simulink model "Assignment_2_simulink_2"  (R2025a)
settings: Solver=FixedStepDiscrete  StartTime=0.0  StopTime=inf  FixedStep=0.1  RelTol=1e-3  EnableMultiTasking=on
values from neighbouring files (symbols this model uses):
  Kv = 0.8    [Assignment_2.m]
  tol = 0.05    [Assignment_2.m]
undefined symbols (not defined in the file or in its folder): angular, linear, v_max
libraries: simulink x4, ros2lib x3
settings Model: Creator=nicola-bertocchi  LastModifiedBy=nicola-bertocchi
settings OptimizationCC: DefaultParameterBehavior=Inlined  EnhancedBackFolding=on  PassReuseOutputArgsAs=Individual arguments  ZeroExternalMemoryAtStartup=off  ZeroInternalMemoryAtStartup=off  MaxStackSize=64  OptimizeBlockOrder=speed  DifferentSizesBufferReuse=on  OptimizationCustomize=off  EfficientTunableParamExpr=on
settings DebuggingCC: ParameterTunabilityLossMsg=error
settings HardwareCC: ProdBitPerLong=64.0  ProdHWDeviceType=Intel->x86-64 (Linux 64)
settings SFSimCC: MATLABDynamicMemAlloc=off
settings RTWCC: SystemTargetFile=ert.tlc  HardwareBoard=Robot Operating System 2 (ROS 2)  TLCOptions="-aInlineSetEventsForThisBaseRateFcn=TLC_FALSE -aSuppressMultiTaskScheduler=TLC_FALSE  -aRateBasedStepFcn=0"  TemplateMakefile=ert_default_tmf  Toolchain=Colcon Tools  TargetLang=C++  Description=Embedded Coder
settings CodeAppCC: ForceParamTrailComments=on  IgnoreCustomStorageClasses=off  OperatorAnnotations=on  SimulinkDataObjDesc=on  SFDataObjDesc=on  InsertBlockDesc=on
settings ERTTargetCC: ExtModeTransport=2.0  ExtModeAutomaticAllocSize=off  RootIOFormat=Structure reference  CodeInterfacePackaging=C++ class

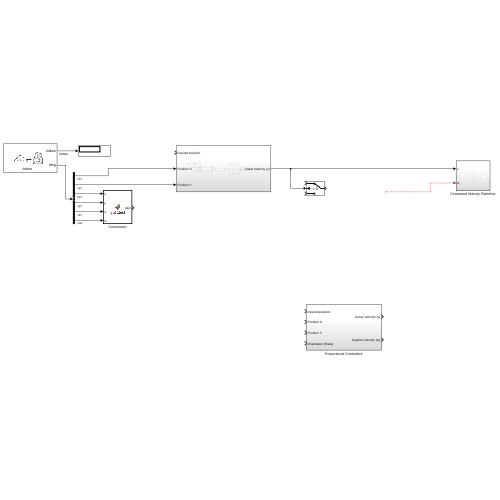
[thumbnail: Simulink's stored preview of the top-level diagram]
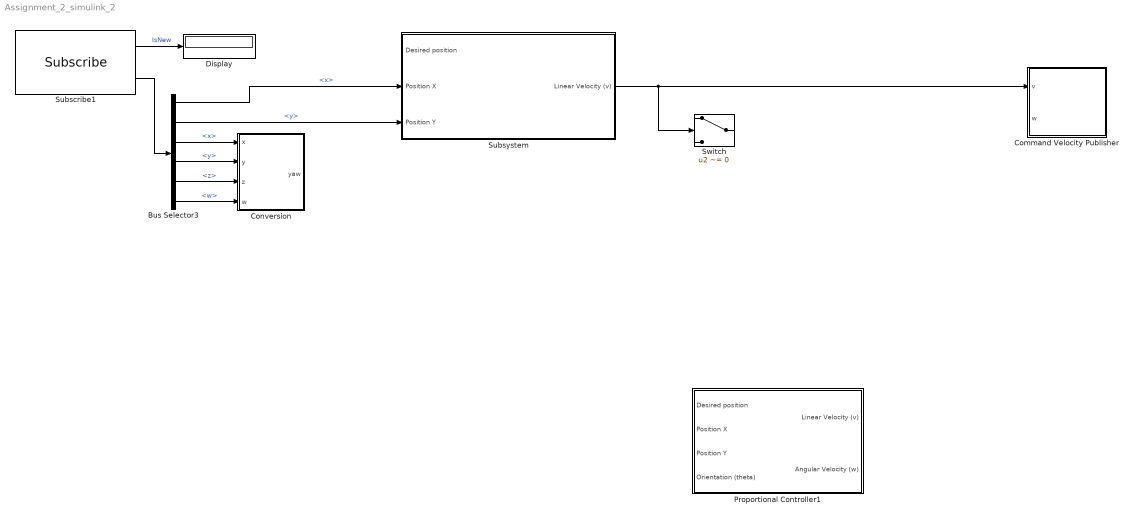
== system Assignment_2_simulink_2 ==
  Bus Selector3 : BusSelector  OutputSignals=pose.pose.position.x,pose.pose.position.y,pose.pose.orientation.x,pose.pose.orientation.y,pose.pose.orientation.z,pose.pose.orientation.w
  Command Velocity Publisher : Subsystem
  Conversion : MATLAB Function  TreatAsAtomicUnit=on
  Display : Display
  Proportional Controller1 : Subsystem
  Subscribe1 : ros2lib/Subscribe  topicSource=Select from ROS network  topic=/odom  messageType=nav_msgs/Odometry  sampleTime=-1  QOSHistory=Keep last  QOSDepth=1  QOSReliability=Reliable  QOSDurability=Volatile  QOSDeadline=Inf  QOSLifespan=Inf  QOSLiveliness=Automatic  QOSLeaseDuration=Inf  QOSAvoidROSNamespaceConventions=off
  Subsystem : Subsystem
  Switch : Switch  Criteria=u2 ~= 0  SaturateOnIntegerOverflow=off  InputSameDT=off
  wires:
  Bus Selector3/6 -> Conversion/4(w)  "<w>"
  Subsystem/1(Linear Velocity (v)) -> Command Velocity Publisher/1(v), Switch/2
  Bus Selector3/1 -> Subsystem/2(Position X)  "<x>"
  Bus Selector3/2 -> Subsystem/3(Position Y)  "<y>"
  Bus Selector3/5 -> Conversion/3(z)  "<z>"
  ? -> Command Velocity Publisher/2(w)
  Subscribe1/2 -> Bus Selector3/1
  Bus Selector3/3 -> Conversion/1(x)  "<x>"
  Bus Selector3/4 -> Conversion/2(y)  "<y>"
  Subscribe1/1 -> Display/1  "IsNew"

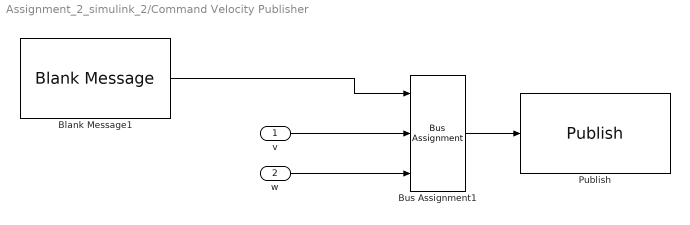
== system Assignment_2_simulink_2/Command Velocity Publisher ==
  v : Inport
  w : Inport  Port=2
  Blank Message1 : ros2lib/Blank Message  messageClass=Message  entityType=geometry_msgs/Twist  messageType=geometry_msgs/Twist  SampleTime=inf
  Bus Assignment1 : BusAssignment  DialogController=Simulink.DDGSource_BusAssignment  AssignedSignals=linear.x,angular.z
  Publish : ros2lib/Publish  topicSource=Specify your own  topic=/cmd_vel  messageType=geometry_msgs/Twist  QOSHistory=Keep last  QOSDepth=1  QOSReliability=Reliable  QOSDurability=Volatile  QOSDeadline=Inf  QOSLifespan=Inf  QOSLiveliness=Automatic  QOSLeaseDuration=Inf  QOSAvoidROSNamespaceConventions=off
  wires:
  Bus Assignment1/1 -> Publish/1
  Blank Message1/1 -> Bus Assignment1/1
  v/1 -> Bus Assignment1/2
  w/1 -> Bus Assignment1/3

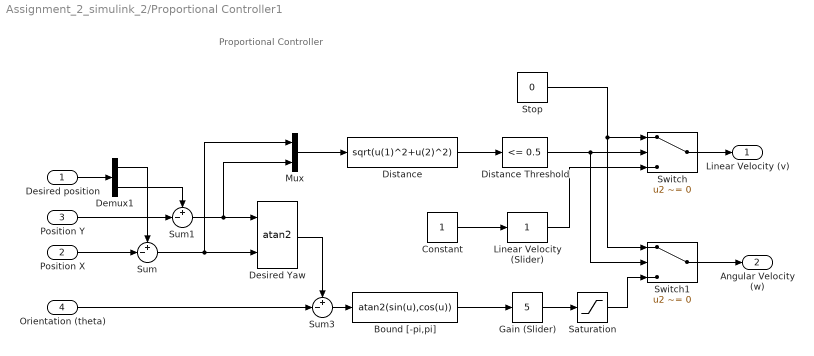
== system Assignment_2_simulink_2/Proportional Controller1 ==
  note: Proportional Controller
  Desired position : Inport
  Position X : Inport  Port=2
  Position Y : Inport  Port=3
  Orientation (theta) : Inport  Port=4
  Bound [-pi,pi] : Fcn  Expr=atan2(sin(u),cos(u))
  Constant : Constant
  Demux1 : Demux  Outputs=2
  Desired Yaw : Trigonometry  Operator=atan2
  Distance : Fcn  Expr=sqrt(u(1)^2+u(2)^2)
  Distance Threshold : simulink/Logic and Bit Operations/Compare To Constant  relop=<=  const=0.5  OutDataTypeStr=boolean
  Gain (Slider) : simulink/Math Operations/Slider Gain  gain=5  low=1  high=10
  Linear Velocity (Slider) : simulink/Math Operations/Slider Gain  gain=1  low=0  high=2
  Mux : Mux  Inputs=2
  Saturation : Saturate
  Stop : Constant  Value=0
  Sum : Sum  Inputs=+-|
  Sum1 : Sum  Inputs=+-|
  Sum3 : Sum  Inputs=+-|
  Switch : Switch  Criteria=u2 ~= 0  SaturateOnIntegerOverflow=off  InputSameDT=off
  Switch1 : Switch  Criteria=u2 ~= 0  SaturateOnIntegerOverflow=off  InputSameDT=off
  Linear Velocity (v) : Outport  VectorParamsAs1DForOutWhenUnconnected=off
  Angular Velocity (w) : Outport  Port=2  VectorParamsAs1DForOutWhenUnconnected=off
  wires:
  Switch1/1 -> Angular Velocity (w)/1
  Linear Velocity (Slider)/1 -> Switch/3
  Switch/1 -> Linear Velocity (v)/1
  Sum3/1 -> Bound [-pi,pi]/1
  Stop/1 -> Switch1/1, Switch/1
  Saturation/1 -> Switch1/3
  Gain (Slider)/1 -> Saturation/1
  Distance Threshold/1 -> Switch1/2, Switch/2
  Sum/1 -> Mux/1, Desired Yaw/2
  Desired Yaw/1 -> Sum3/1
  Orientation (theta)/1 -> Sum3/2
  Bound [-pi,pi]/1 -> Gain (Slider)/1
  Mux/1 -> Distance/1
  Distance/1 -> Distance Threshold/1
  Position X/1 -> Sum/2
  Position Y/1 -> Sum1/2
  Desired position/1 -> Demux1/1
  Constant/1 -> Linear Velocity (Slider)/1
  Sum1/1 -> Mux/2, Desired Yaw/1
  Demux1/2 -> Sum1/1
  Demux1/1 -> Sum/1

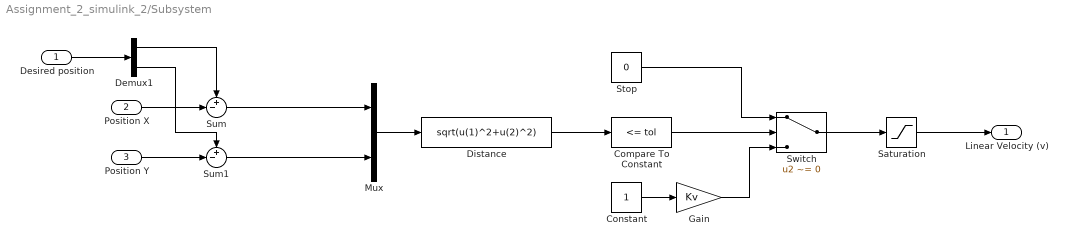
== system Assignment_2_simulink_2/Subsystem ==
  Desired position : Inport
  Position X : Inport  Port=2
  Position Y : Inport  Port=3
  Compare To Constant : simulink/Logic and Bit Operations/Compare To Constant  relop=<=  const=tol  OutDataTypeStr=boolean
  Constant : Constant
  Demux1 : Demux  Outputs=2
  Distance : Fcn  Expr=sqrt(u(1)^2+u(2)^2)
  Gain : Gain  Gain=Kv
  Mux : Mux  Inputs=2
  Saturation : Saturate  UpperLimit=v_max  LowerLimit=0
  Stop : Constant  Value=0
  Sum : Sum  Inputs=+-|
  Sum1 : Sum  Inputs=+-|
  Switch : Switch  Criteria=u2 ~= 0  SaturateOnIntegerOverflow=off  InputSameDT=off
  Linear Velocity (v) : Outport  VectorParamsAs1DForOutWhenUnconnected=off
  wires:
  Constant/1 -> Gain/1
  Gain/1 -> Switch/3
  Position Y/1 -> Sum1/2
  Sum/1 -> Mux/1
  Saturation/1 -> Linear Velocity (v)/1
  Demux1/2 -> Sum1/1
  Position X/1 -> Sum/2
  Mux/1 -> Distance/1
  Desired position/1 -> Demux1/1
  Compare To Constant/1 -> Switch/2
  Distance/1 -> Compare To Constant/1
  Switch/1 -> Saturation/1
  Demux1/1 -> Sum/1
  Sum1/1 -> Mux/2
  Stop/1 -> Switch/1

== matlab function Assignment_2_simulink_2/Conversion ==
  data: yaw output; x input; y input; z input; w input
function yaw  = quat2eul(x,y,z,w)
%#codegen

% Convert the quaternion to a yaw angle (zyx euler angle)
eul = quat2eul([w,x,y,z]);
yaw = eul(1);

end
